simulink model "kinSwCtrl_v2_3"  (R2015a)
settings: Solver=ode45  StartTime=0.0  StopTime=t_sim  RelTol=1e-3
InitFcn:
  | set_kinSwCtrl_v2_2;
StopFcn:
  | plot_kinSwCtrl2;
values from neighbouring files (symbols this model uses):
  alpha_0 = 120*pi/180    (= 2.09439510239)    [set_kinSwCtrl_v2.m]    (also in set_kinSwCtrl_v2_2.m)
  alpha_min = 90*pi/180    (= 1.57079632679)    [set_kinSwCtrl_v2.m]    (also in set_kinSwCtrl_v2_2.m = 1.3962634016)
  alpha_tgt = 70*pi/180    (= 1.2217304764)    [set_kinSwCtrl_v2_2.m]
  l_min = 0.7    [set_kinSwCtrl_v2.m]    (also in set_kinSwCtrl_v2_2.m)
  l_tgt = 0.9    [set_kinSwCtrl_v2_2.m]
  v_alpha = (alpha_min-alpha_0)/t_sim    (= -0.523598775598)    [set_kinSwCtrl_v2.m]    (also in set_kinSwCtrl_v2_2.m = -0.436332312999)
libraries: simulink x1
settings Model: Creator=smsong  LastModifiedBy=smsong

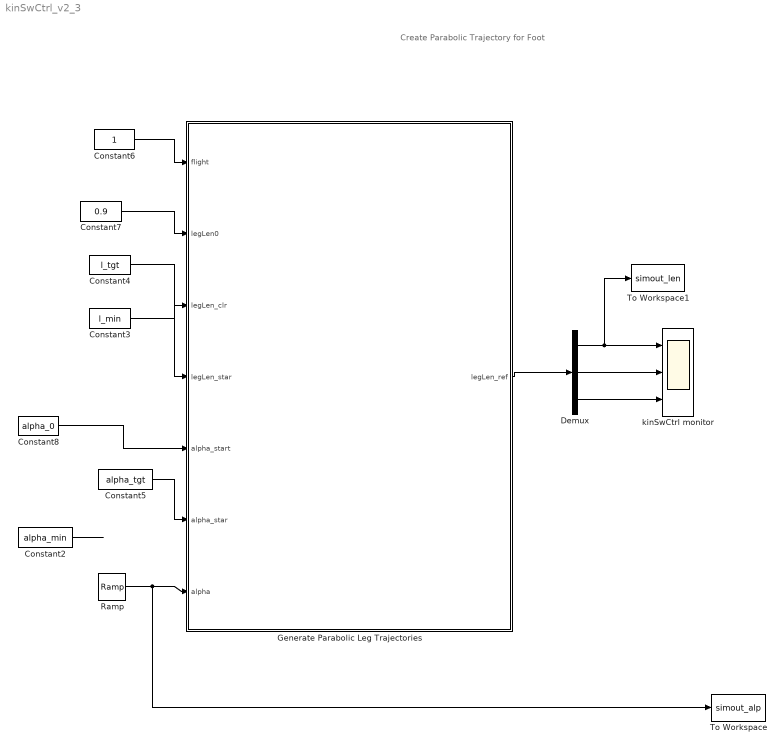
== system kinSwCtrl_v2_3 ==
  note: Create Parabolic
      | Trajectory for Foot
  Constant2 : Constant  Value=alpha_min
  Constant3 : Constant  Value=l_min
  Constant4 : Constant  Value=l_tgt
  Constant5 : Constant  Value=alpha_tgt
  Constant6 : Constant
  Constant7 : Constant  Value=0.9
  Constant8 : Constant  Value=alpha_0
  Demux : Demux  Outputs=3
  Generate Parabolic Leg Trajectories : MATLAB Function  TreatAsAtomicUnit=on
  Ramp : simulink/Sources/Ramp  slope=v_alpha  start=0  X0=alpha_0
  To Workspace : ToWorkspace  VariableName=simout_alp  SaveFormat=Structure With Time  SampleTime=-1
  To Workspace1 : ToWorkspace  VariableName=simout_len  SaveFormat=Structure With Time  SampleTime=-1
  kinSwCtrl monitor : Scope  NumInputPorts=3
      settings: YMin=-0.1~-0.1~-0.1  YMax=1.1~1.1~1.1  SaveName=ScopeData13
  wires:
  Constant6/1 -> Generate Parabolic Leg Trajectories/1(flight)
  Constant7/1 -> Generate Parabolic Leg Trajectories/2(legLen0)
  Constant4/1 -> Generate Parabolic Leg Trajectories/4(legLen_star)
  Constant3/1 -> Generate Parabolic Leg Trajectories/3(legLen_clr)
  Constant5/1 -> Generate Parabolic Leg Trajectories/6(alpha_star)
  Ramp/1 -> To Workspace/1, Generate Parabolic Leg Trajectories/7(alpha)
  Generate Parabolic Leg Trajectories/1(legLen_ref) -> Demux/1
  Demux/1 -> kinSwCtrl monitor/1, To Workspace1/1
  Demux/2 -> kinSwCtrl monitor/2
  Demux/3 -> kinSwCtrl monitor/3
  Constant2/1 -> ?
  Constant8/1 -> Generate Parabolic Leg Trajectories/5(alpha_start)

== matlab function kinSwCtrl_v2_3/Generate Parabolic Leg Trajectories ==
  data: legLen_ref output size=3; flight input; legLen0 input; legLen_clr input; legLen_star input; alpha_start input; alpha_star input; alpha input
%% Parabolic trajectory generation for leg angle and length
% est_duration: estimated flight time
% time_remaining: time until estimated touchdown
% legAlp0: legAlp at takeoff
%   legAlp is the angle of attack
% legLen0: legLen at takeoff
% legAlp_star: desired legAlp
% legLen_star: desired legLen
% legLen_min: min legLen for ground clearance
% min_f_duration: minimum trajectory time

function legLen_ref   =  ...
          GenerateReferenceLegLength(flight, ...
                    legLen0, legLen_clr, legLen_star,   ...
                    alpha_start, alpha_star, alpha)

if ~flight
    legLen_ref = [0.9;0;0];
    return;
end

    
  % split duration into thirds.  First segment: parabola from legLen0 to
  % legLen_min.  Second and third segments, cos to landing.
  alpha_d   = abs(alpha_star-alpha_start);
  alpha_r   = max(abs(alpha_star-alpha), 0);
  da3 = alpha_d / 3;
  if alpha_r > 2*da3;
    legLen_star_a = legLen_clr + (legLen0-legLen_clr)*((alpha_r-2*da3)/da3)^2;
    dlegLen_star_a = -(legLen0-legLen_clr)*2*(alpha_r-2*da3)/da3/da3;
    ddlegLen_star_a = (legLen0-legLen_clr)*2/da3^2;
  else
    legLen_star_a = legLen_star + (legLen_clr-legLen_star)/2*(1-cos(alpha_r/(2*da3)*pi));
    dlegLen_star_a = -(legLen_clr-legLen_star)/2*sin(alpha_r/(2*da3)*pi)*pi/(2*da3);
    ddlegLen_star_a = (legLen_clr-legLen_star)/2*cos(alpha_r/(2*da3)*pi)*(pi/(2*da3))^2;
  end
  
  % track a sinusoidal z of amplitude max_retract, finishing a half-cycle by t_end
  legLen_ref = [legLen_star_a; dlegLen_star_a; ddlegLen_star_a];
